simulink model "SS_Servo_LP"  (R2019b)
settings: Solver=VariableStepAuto  StartTime=0.0  StopTime=60  RelTol=1e-3
undefined symbols (not defined in the file): Servo_LP_den, Servo_LP_num
settings Model: Creator=toons  LastModifiedBy=toons

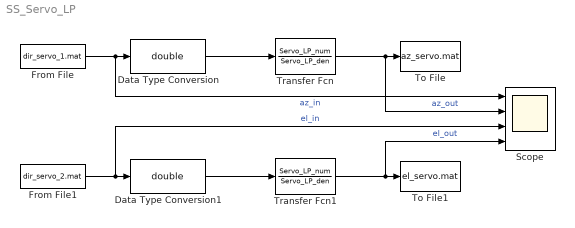
== system SS_Servo_LP ==
  Data Type Conversion : DataTypeConversion  OutDataTypeStr=double
  Data Type Conversion1 : DataTypeConversion  OutDataTypeStr=double
  From File : FromFile  FileName=dir_servo_1.mat  SampleTime=0.001
  From File1 : FromFile  FileName=dir_servo_2.mat  SampleTime=0.001
  Scope : Scope  NumInputPorts=4
  To File : ToFile  Filename=az_servo.mat  SaveFormat=Timeseries
  To File1 : ToFile  Filename=el_servo.mat  SaveFormat=Timeseries
  Transfer Fcn : TransferFcn  Numerator=Servo_LP_num  Denominator=Servo_LP_den
  Transfer Fcn1 : TransferFcn  Numerator=Servo_LP_num  Denominator=Servo_LP_den
  wires:
  From File/1 -> Scope/1, Data Type Conversion/1  "az_in"
  From File1/1 -> Scope/3, Data Type Conversion1/1  "el_in"
  Data Type Conversion1/1 -> Transfer Fcn1/1
  Transfer Fcn1/1 -> Scope/4, To File1/1  "el_out"
  Transfer Fcn/1 -> Scope/2, To File/1  "az_out"
  Data Type Conversion/1 -> Transfer Fcn/1
